simulink model "SF013A_PullCmpActv"  (R2013b)
settings: Solver=FixedStepDiscrete  SolverMode=SingleTasking  StartTime=0.0  StopTime=1  FixedStep=0.002  RelTol=1e-3
values from neighbouring files (symbols this model uses):
  ARCHGLBPRM_100MILLISEC_SEC_F32 = DataDict.Constant    [SF013A_PullCmpActv_DataDict.m]
  ARCHGLBPRM_2MILLISEC_SEC_F32 = DataDict.Constant    [SF013A_PullCmpActv_DataDict.m]
  ARCHGLBPRM_FLOATZEROTHD_ULS_F32 = DataDict.Constant    [SF013A_PullCmpActv_DataDict.m]
  INTGTRSCARSHOTERM_ULS_F32 = DataDict.Constant    [SF013A_PullCmpActv_DataDict.m]
  LONGTERMINTGTRSCAR_ULS_F32 = DataDict.Constant    [SF013A_PullCmpActv_DataDict.m]
  MICROSECTOSEC_ULS_F32 = DataDict.Constant    [SF013A_PullCmpActv_DataDict.m]
  MINSTOSEC_SECPERMINS_F32 = DataDict.Constant    [SF013A_PullCmpActv_DataDict.m]
  PullCmpActvCmpLrnTiDecShoTerm = DataDict.Calibration    [SF013A_PullCmpActv_DataDict.m]
  PullCmpActvCmpLrnTiIncShoTerm = DataDict.Calibration    [SF013A_PullCmpActv_DataDict.m]
  PullCmpActvCmpLrnTiLongTerm = DataDict.Calibration    [SF013A_PullCmpActv_DataDict.m]
  PullCmpActvCmpShoTermRstHwAgThd = DataDict.Calibration    [SF013A_PullCmpActv_DataDict.m]
  PullCmpActvCmpShoTermRstHwTqThd = DataDict.Calibration    [SF013A_PullCmpActv_DataDict.m]
  PullCmpActvCmpShoTermRstLatAThd = DataDict.Calibration    [SF013A_PullCmpActv_DataDict.m]
  PullCmpActvCmpShoTermRstYawRateThd = DataDict.Calibration    [SF013A_PullCmpActv_DataDict.m]
  PullCmpActvEna = DataDict.Calibration    [SF013A_PullCmpActv_DataDict.m]
  PullCmpActvLongTermLim = DataDict.Calibration    [SF013A_PullCmpActv_DataDict.m]
  PullCmpActvLrngEnaAgConfMinMgn = DataDict.Calibration    [SF013A_PullCmpActv_DataDict.m]
  PullCmpActvLrngEnaHwAgMaxMgn = DataDict.Calibration    [SF013A_PullCmpActv_DataDict.m]
  PullCmpActvLrngEnaHwTqMaxMgn = DataDict.Calibration    [SF013A_PullCmpActv_DataDict.m]
  PullCmpActvLrngEnaHwVelMaxMgn = DataDict.Calibration    [SF013A_PullCmpActv_DataDict.m]
  PullCmpActvLrngEnaLatAMaxMgn = DataDict.Calibration    [SF013A_PullCmpActv_DataDict.m]
  PullCmpActvLrngEnaTiThd = DataDict.Calibration    [SF013A_PullCmpActv_DataDict.m]
  PullCmpActvLrngEnaVehSpdMaxMgn = DataDict.Calibration    [SF013A_PullCmpActv_DataDict.m]
  PullCmpActvLrngEnaVehSpdMinMgn = DataDict.Calibration    [SF013A_PullCmpActv_DataDict.m]
  PullCmpActvLrngEnaVehSpdRateMaxMgn = DataDict.Calibration    [SF013A_PullCmpActv_DataDict.m]
  PullCmpActvLrngEnaYawRateMaxMgn = DataDict.Calibration    [SF013A_PullCmpActv_DataDict.m]
  PullCmpActvOpstSignTiShoTerm = DataDict.Calibration    [SF013A_PullCmpActv_DataDict.m]
  PullCmpActvOutpMaxRate = DataDict.Calibration    [SF013A_PullCmpActv_DataDict.m]
  PullCmpActvPullCmpShoTermLim = DataDict.Calibration    [SF013A_PullCmpActv_DataDict.m]
  PullCmpActvPullCmpTotLim = DataDict.Calibration    [SF013A_PullCmpActv_DataDict.m]
  PullCmpActvPullErrLimLongTerm = DataDict.Calibration    [SF013A_PullCmpActv_DataDict.m]
  PullCmpActvPullErrMgnThd = DataDict.Calibration    [SF013A_PullCmpActv_DataDict.m]
  PullCmpActvPullErrShoTermLim = DataDict.Calibration    [SF013A_PullCmpActv_DataDict.m]
  PullCmpActvShoTermRampTi = DataDict.Calibration    [SF013A_PullCmpActv_DataDict.m]
  SysGlbPrmSysTqRat = DataDict.ImprtdCal    [SF013A_PullCmpActv_DataDict.m]
libraries: NxtrAbslt x9, Fil x8, simulink x7, NxtrLim x6, FixdToFloat x3, NxtrSign x3, NxtrMin x3, NxtrNvM x2, NxtrMax x2, FloatToFixd x1, LnrIntrpn x1
(part 3 of 4)

== system SF013A_PullCmpActv/PullCmpActv/PullCmpActvPer1/PullCmpActvPer1/ActvCmpEna/ElapsedTime/If not true elapsed time = 0 ==
  Action Port : ActionPort  ActionType=then
  Constant : Constant  Value=0  OutDataTypeStr=single
  CopyRight2 : Subsystem  Description=|  mask(Copyright Information){none=on}
      | Copyright info block.                                               
      |                                                                     
      | Place copyright information at the top of every subsystem in design.
      mask prompts: none "No parameters"
      mask help: Place copyright information at the top of every subsystem in design.
      mask Display:
      | NxtrConf = 'Nexteer Confidential';
      | 
      | sys = bdroot; %handle for the current model ("system")
      | first = get_param(sys,'Created');
      | if(isempty(first))
      |     first = datestr(now,'yyyy');
      | else
      |     first = first(end-3:end);  %year is last four digits
      | end
      | 
      | last = get_param(sys,'LastModifiedDate');
      | if isempty(last)
      |     last = datestr(now,'yyyy');
      | else
      |     last = last(end-3:end);
      | end
      | 
      | if strcmp(first,last)
      |     fprintf('%s -- Copyright %s Nexteer',NxtrConf,first)
      | else
      |     fprintf('%s -- %s%s- %s Nexteer',NxtrConf,char(169),first,last)
      | end
  SpanTi : Outport
  wires:
  Constant/1 -> SpanTi/1

== system SF013A_PullCmpActv/PullCmpActv/PullCmpActvPer1/PullCmpActvPer1/ActvCmpEna/ElapsedTime/If true and last step is true calculate elapsed time  ==
  Action Port : ActionPort  ActionType=else
  Constant1 : Constant  Value=MICROSECTOSEC_ULS_F32
  CopyRight2 : Subsystem  Description=|  mask(Copyright Information){none=on}
      | Copyright info block.                                               
      |                                                                     
      | Place copyright information at the top of every subsystem in design.
      mask prompts: none "No parameters"
      mask help: Place copyright information at the top of every subsystem in design.
      mask Display:
      | NxtrConf = 'Nexteer Confidential';
      | 
      | sys = bdroot; %handle for the current model ("system")
      | first = get_param(sys,'Created');
      | if(isempty(first))
      |     first = datestr(now,'yyyy');
      | else
      |     first = first(end-3:end);  %year is last four digits
      | end
      | 
      | last = get_param(sys,'LastModifiedDate');
      | if isempty(last)
      |     last = datestr(now,'yyyy');
      | else
      |     last = last(end-3:end);
      | end
      | 
      | if strcmp(first,last)
      |     fprintf('%s -- Copyright %s Nexteer',NxtrConf,first)
      | else
      |     fprintf('%s -- %s%s- %s Nexteer',NxtrConf,char(169),first,last)
      | end
  Data Store Read : DataStoreRead  DataStoreName=RefTiEnaLrng
  Divide : Product  Inputs=**
  FixdToFloat_f32_u32 : FixdToFloat/FixdToFloat_f32_u32  Param1=0
  GetTiSpan100MicroSec32bit : Subsystem
  SpanTi : Outport
  wires:
  Constant1/1 -> Divide/2
  Divide/1 -> SpanTi/1
  GetTiSpan100MicroSec32bit/1(TiSpan) -> FixdToFloat_f32_u32/1
  Data Store Read/1 -> GetTiSpan100MicroSec32bit/1(RefTmr)
  FixdToFloat_f32_u32/1 -> Divide/1

== system SF013A_PullCmpActv/PullCmpActv/PullCmpActvPer1/PullCmpActvPer1/ActvCmpEna/ElapsedTime/If true and last step not true elapsed time = 0 get reference time  ==
  Action Port : ActionPort  ActionType=elseif
  Constant : Constant  Value=0  OutDataTypeStr=single
  CopyRight2 : Subsystem  Description=|  mask(Copyright Information){none=on}
      | Copyright info block.                                               
      |                                                                     
      | Place copyright information at the top of every subsystem in design.
      mask prompts: none "No parameters"
      mask help: Place copyright information at the top of every subsystem in design.
      mask Display:
      | NxtrConf = 'Nexteer Confidential';
      | 
      | sys = bdroot; %handle for the current model ("system")
      | first = get_param(sys,'Created');
      | if(isempty(first))
      |     first = datestr(now,'yyyy');
      | else
      |     first = first(end-3:end);  %year is last four digits
      | end
      | 
      | last = get_param(sys,'LastModifiedDate');
      | if isempty(last)
      |     last = datestr(now,'yyyy');
      | else
      |     last = last(end-3:end);
      | end
      | 
      | if strcmp(first,last)
      |     fprintf('%s -- Copyright %s Nexteer',NxtrConf,first)
      | else
      |     fprintf('%s -- %s%s- %s Nexteer',NxtrConf,char(169),first,last)
      | end
  Data Store Write : DataStoreWrite  DataStoreName=RefTiEnaLrng
  GetRefTmr100MicroSec32bit : Subsystem
  "SpanTi " : Outport
  wires:
  Constant/1 -> "SpanTi "/1
  GetRefTmr100MicroSec32bit/1(RefTmr) -> Data Store Write/1

== system SF013A_PullCmpActv/PullCmpActv/PullCmpActvPer1/PullCmpActvPer1/Calc_CmpTot/If Action Subsystem/CopyRight2 ==

== system SF013A_PullCmpActv/PullCmpActv/PullCmpActvPer1/PullCmpActvPer1/Calc_CmpTot/If Action Subsystem1/CopyRight2 ==

== system SF013A_PullCmpActv/PullCmpActv/PullCmpActvPer1/PullCmpActvPer1/ShoTermCmp/CalcIntgtrGain /CopyRight2 ==

== system SF013A_PullCmpActv/PullCmpActv/PullCmpActvPer1/PullCmpActvPer1/ShoTermCmp/CalcIntgtrGain /ElapsedTime ==
  note: If
  "OpstSign " : Inport
  CopyRight2 : Subsystem  Description=|  mask(Copyright Information){none=on}
      | Copyright info block.                                               
      |                                                                     
      | Place copyright information at the top of every subsystem in design.
      mask prompts: none "No parameters"
      mask help: Place copyright information at the top of every subsystem in design.
      mask Display:
      | NxtrConf = 'Nexteer Confidential';
      | 
      | sys = bdroot; %handle for the current model ("system")
      | first = get_param(sys,'Created');
      | if(isempty(first))
      |     first = datestr(now,'yyyy');
      | else
      |     first = first(end-3:end);  %year is last four digits
      | end
      | 
      | last = get_param(sys,'LastModifiedDate');
      | if isempty(last)
      |     last = datestr(now,'yyyy');
      | else
      |     last = last(end-3:end);
      | end
      | 
      | if strcmp(first,last)
      |     fprintf('%s -- Copyright %s Nexteer',NxtrConf,first)
      | else
      |     fprintf('%s -- %s%s- %s Nexteer',NxtrConf,char(169),first,last)
      | end
  Data Store Read : DataStoreRead  Priority=1  DataStoreName=OpstSignPrev
      settings: AttributesFormatString=priority: %<Priority>
  Data Store Write : DataStoreWrite  Priority=2  DataStoreName=OpstSignPrev
      settings: AttributesFormatString="priority:  %<Priority>"
  If : If  NumInputs=2  IfExpression=u1  ElseIfExpressions=u2
  If not true elapsed time = 0 : Subsystem  TreatAsAtomicUnit=on
  "If true and last step is true calculate elapsed time " : Subsystem  TreatAsAtomicUnit=on
  "If true and last step not true elapsed time = 0 get reference time " : Subsystem  TreatAsAtomicUnit=on
  Logical Operator : Logic  AllPortsSameDT=off  OutDataTypeStr=boolean
  Logical Operator1 : Logic  Operator=NOT  AllPortsSameDT=off  OutDataTypeStr=boolean
  Logical Operator2 : Logic  Operator=NOT  AllPortsSameDT=off  OutDataTypeStr=boolean
  Merge : Merge  Inputs=3
  ElapsedTime : Outport
  wires:
  If/1 -> If not true elapsed time = 0/Action
  If/2 -> "If true and last step not true elapsed time = 0 get reference time "/Action
  If/3 -> "If true and last step is true calculate elapsed time "/Action
  If not true elapsed time = 0/1(SpanTi) -> Merge/1
  "If true and last step not true elapsed time = 0 get reference time "/1("SpanTi ") -> Merge/2
  "If true and last step is true calculate elapsed time "/1(SpanTi) -> Merge/3
  Merge/1 -> ElapsedTime/1
  "OpstSign "/1 -> Logical Operator2/1, Logical Operator/1, Data Store Write/1
  Logical Operator1/1 -> Logical Operator/2
  Data Store Read/1 -> Logical Operator1/1
  Logical Operator/1 -> If/2
  Logical Operator2/1 -> If/1

== system SF013A_PullCmpActv/PullCmpActv/PullCmpActvPer1/PullCmpActvPer1/ShoTermCmp/CalcIntgtrGain /If Action Subsystem ==
  In1 : Inport
  Action Port : ActionPort  ActionType=then
  CopyRight2 : Subsystem  Description=|  mask(Copyright Information){none=on}
      | Copyright info block.                                               
      |                                                                     
      | Place copyright information at the top of every subsystem in design.
      mask prompts: none "No parameters"
      mask help: Place copyright information at the top of every subsystem in design.
      mask Display:
      | NxtrConf = 'Nexteer Confidential';
      | 
      | sys = bdroot; %handle for the current model ("system")
      | first = get_param(sys,'Created');
      | if(isempty(first))
      |     first = datestr(now,'yyyy');
      | else
      |     first = first(end-3:end);  %year is last four digits
      | end
      | 
      | last = get_param(sys,'LastModifiedDate');
      | if isempty(last)
      |     last = datestr(now,'yyyy');
      | else
      |     last = last(end-3:end);
      | end
      | 
      | if strcmp(first,last)
      |     fprintf('%s -- Copyright %s Nexteer',NxtrConf,first)
      | else
      |     fprintf('%s -- %s%s- %s Nexteer',NxtrConf,char(169),first,last)
      | end
  Out1 : Outport
  wires:
  In1/1 -> Out1/1

== system SF013A_PullCmpActv/PullCmpActv/PullCmpActvPer1/PullCmpActvPer1/ShoTermCmp/CalcIntgtrGain /If Action Subsystem1 ==
  In1 : Inport
  Action Port : ActionPort  ActionType=else
  CopyRight2 : Subsystem  Description=|  mask(Copyright Information){none=on}
      | Copyright info block.                                               
      |                                                                     
      | Place copyright information at the top of every subsystem in design.
      mask prompts: none "No parameters"
      mask help: Place copyright information at the top of every subsystem in design.
      mask Display:
      | NxtrConf = 'Nexteer Confidential';
      | 
      | sys = bdroot; %handle for the current model ("system")
      | first = get_param(sys,'Created');
      | if(isempty(first))
      |     first = datestr(now,'yyyy');
      | else
      |     first = first(end-3:end);  %year is last four digits
      | end
      | 
      | last = get_param(sys,'LastModifiedDate');
      | if isempty(last)
      |     last = datestr(now,'yyyy');
      | else
      |     last = last(end-3:end);
      | end
      | 
      | if strcmp(first,last)
      |     fprintf('%s -- Copyright %s Nexteer',NxtrConf,first)
      | else
      |     fprintf('%s -- %s%s- %s Nexteer',NxtrConf,char(169),first,last)
      | end
  Out1 : Outport
  wires:
  In1/1 -> Out1/1

== system SF013A_PullCmpActv/PullCmpActv/PullCmpActvPer1/PullCmpActvPer1/ShoTermCmp/CalcIntgtrGain /If Action Subsystem2 ==
  CmpLrnTi_Dec_ShoTerm : Inport
  Action Port : ActionPort  ActionType=then
  Constant3 : Constant  Value=INTGTRSCARSHOTERM_ULS_F32
  Constant4 : Constant  Value=ARCHGLBPRM_2MILLISEC_SEC_F32
  CopyRight2 : Subsystem  Description=|  mask(Copyright Information){none=on}
      | Copyright info block.                                               
      |                                                                     
      | Place copyright information at the top of every subsystem in design.
      mask prompts: none "No parameters"
      mask help: Place copyright information at the top of every subsystem in design.
      mask Display:
      | NxtrConf = 'Nexteer Confidential';
      | 
      | sys = bdroot; %handle for the current model ("system")
      | first = get_param(sys,'Created');
      | if(isempty(first))
      |     first = datestr(now,'yyyy');
      | else
      |     first = first(end-3:end);  %year is last four digits
      | end
      | 
      | last = get_param(sys,'LastModifiedDate');
      | if isempty(last)
      |     last = datestr(now,'yyyy');
      | else
      |     last = last(end-3:end);
      | end
      | 
      | if strcmp(first,last)
      |     fprintf('%s -- Copyright %s Nexteer',NxtrConf,first)
      | else
      |     fprintf('%s -- %s%s- %s Nexteer',NxtrConf,char(169),first,last)
      | end
  Data Store Write : DataStoreWrite  DataStoreName=IntgtrGainDecShoTerm
  Data Store Write1 : DataStoreWrite  DataStoreName=CmpLrnTiDecShoTerm
  Divide : Product  Inputs=*/
  Product : Product
  CmpIntglGain_Dec_ShoTerm : Outport
  wires:
  Constant3/1 -> Divide/1
  Product/1 -> CmpIntglGain_Dec_ShoTerm/1, Data Store Write/1
  Constant4/1 -> Product/1
  Divide/1 -> Product/2
  CmpLrnTi_Dec_ShoTerm/1 -> Data Store Write1/1, Divide/2

== system SF013A_PullCmpActv/PullCmpActv/PullCmpActvPer1/PullCmpActvPer1/ShoTermCmp/CalcIntgtrGain /If Action Subsystem3 ==
  In1 : Inport
  Action Port : ActionPort  ActionType=else
  CopyRight2 : Subsystem  Description=|  mask(Copyright Information){none=on}
      | Copyright info block.                                               
      |                                                                     
      | Place copyright information at the top of every subsystem in design.
      mask prompts: none "No parameters"
      mask help: Place copyright information at the top of every subsystem in design.
      mask Display:
      | NxtrConf = 'Nexteer Confidential';
      | 
      | sys = bdroot; %handle for the current model ("system")
      | first = get_param(sys,'Created');
      | if(isempty(first))
      |     first = datestr(now,'yyyy');
      | else
      |     first = first(end-3:end);  %year is last four digits
      | end
      | 
      | last = get_param(sys,'LastModifiedDate');
      | if isempty(last)
      |     last = datestr(now,'yyyy');
      | else
      |     last = last(end-3:end);
      | end
      | 
      | if strcmp(first,last)
      |     fprintf('%s -- Copyright %s Nexteer',NxtrConf,first)
      | else
      |     fprintf('%s -- %s%s- %s Nexteer',NxtrConf,char(169),first,last)
      | end
  Out1 : Outport
  wires:
  In1/1 -> Out1/1

== system SF013A_PullCmpActv/PullCmpActv/PullCmpActvPer1/PullCmpActvPer1/ShoTermCmp/CalcIntgtrGain /If Action Subsystem4 ==
  CmpLrnTi_Inc_ShoTerm : Inport
  Action Port : ActionPort  ActionType=then
  Constant3 : Constant  Value=INTGTRSCARSHOTERM_ULS_F32
  Constant4 : Constant  Value=ARCHGLBPRM_2MILLISEC_SEC_F32
  CopyRight2 : Subsystem  Description=|  mask(Copyright Information){none=on}
      | Copyright info block.                                               
      |                                                                     
      | Place copyright information at the top of every subsystem in design.
      mask prompts: none "No parameters"
      mask help: Place copyright information at the top of every subsystem in design.
      mask Display:
      | NxtrConf = 'Nexteer Confidential';
      | 
      | sys = bdroot; %handle for the current model ("system")
      | first = get_param(sys,'Created');
      | if(isempty(first))
      |     first = datestr(now,'yyyy');
      | else
      |     first = first(end-3:end);  %year is last four digits
      | end
      | 
      | last = get_param(sys,'LastModifiedDate');
      | if isempty(last)
      |     last = datestr(now,'yyyy');
      | else
      |     last = last(end-3:end);
      | end
      | 
      | if strcmp(first,last)
      |     fprintf('%s -- Copyright %s Nexteer',NxtrConf,first)
      | else
      |     fprintf('%s -- %s%s- %s Nexteer',NxtrConf,char(169),first,last)
      | end
  Data Store Write : DataStoreWrite  DataStoreName=CmpLrnTiIncShoTerm
  Data Store Write1 : DataStoreWrite  DataStoreName=IntgtrGainIncShoTerm
  Divide : Product  Inputs=*/
  Product : Product
  CmpIntglGain_Inc_ShoTerm : Outport
  wires:
  CmpLrnTi_Inc_ShoTerm/1 -> Data Store Write/1, Divide/2
  Divide/1 -> Product/2
  Constant4/1 -> Product/1
  Constant3/1 -> Divide/1
  Product/1 -> CmpIntglGain_Inc_ShoTerm/1, Data Store Write1/1

== system SF013A_PullCmpActv/PullCmpActv/PullCmpActvPer1/PullCmpActvPer1/ShoTermCmp/CalcIntgtrGain /If Action Subsystem5 ==
  In1 : Inport
  Action Port : ActionPort  ActionType=else
  CopyRight2 : Subsystem  Description=|  mask(Copyright Information){none=on}
      | Copyright info block.                                               
      |                                                                     
      | Place copyright information at the top of every subsystem in design.
      mask prompts: none "No parameters"
      mask help: Place copyright information at the top of every subsystem in design.
      mask Display:
      | NxtrConf = 'Nexteer Confidential';
      | 
      | sys = bdroot; %handle for the current model ("system")
      | first = get_param(sys,'Created');
      | if(isempty(first))
      |     first = datestr(now,'yyyy');
      | else
      |     first = first(end-3:end);  %year is last four digits
      | end
      | 
      | last = get_param(sys,'LastModifiedDate');
      | if isempty(last)
      |     last = datestr(now,'yyyy');
      | else
      |     last = last(end-3:end);
      | end
      | 
      | if strcmp(first,last)
      |     fprintf('%s -- Copyright %s Nexteer',NxtrConf,first)
      | else
      |     fprintf('%s -- %s%s- %s Nexteer',NxtrConf,char(169),first,last)
      | end
  Out1 : Outport
  wires:
  In1/1 -> Out1/1

== system SF013A_PullCmpActv/PullCmpActv/PullCmpActvPer1/PullCmpActvPer1/ShoTermCmp/ErrIntgtr & ActvLim /CopyRight2 ==

== system SF013A_PullCmpActv/PullCmpActv/PullCmpActvPer1/PullCmpActvPer1/ShoTermCmp/ErrIntgtr & ActvLim /If Action Subsystem2 ==
  In1 : Inport
  Action Port : ActionPort  ActionType=then
  CopyRight2 : Subsystem  Description=|  mask(Copyright Information){none=on}
      | Copyright info block.                                               
      |                                                                     
      | Place copyright information at the top of every subsystem in design.
      mask prompts: none "No parameters"
      mask help: Place copyright information at the top of every subsystem in design.
      mask Display:
      | NxtrConf = 'Nexteer Confidential';
      | 
      | sys = bdroot; %handle for the current model ("system")
      | first = get_param(sys,'Created');
      | if(isempty(first))
      |     first = datestr(now,'yyyy');
      | else
      |     first = first(end-3:end);  %year is last four digits
      | end
      | 
      | last = get_param(sys,'LastModifiedDate');
      | if isempty(last)
      |     last = datestr(now,'yyyy');
      | else
      |     last = last(end-3:end);
      | end
      | 
      | if strcmp(first,last)
      |     fprintf('%s -- Copyright %s Nexteer',NxtrConf,first)
      | else
      |     fprintf('%s -- %s%s- %s Nexteer',NxtrConf,char(169),first,last)
      | end
  Out1 : Outport
  wires:
  In1/1 -> Out1/1

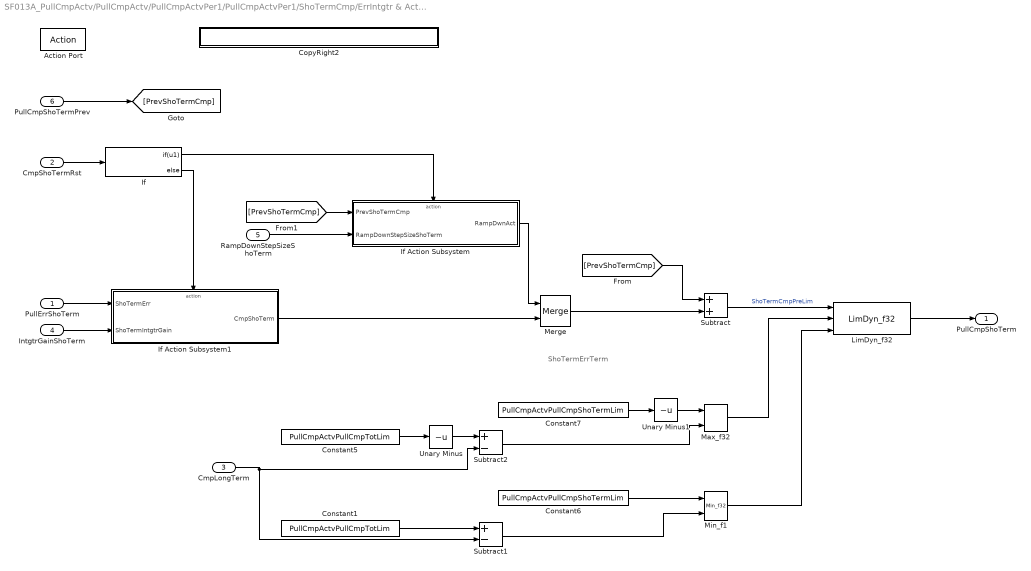
== system SF013A_PullCmpActv/PullCmpActv/PullCmpActvPer1/PullCmpActvPer1/ShoTermCmp/ErrIntgtr & ActvLim /If Action Subsystem3 ==
  note: ShoTermErrTerm
  PullErrShoTerm : Inport
  "CmpShoTermRst " : Inport  Port=2
  CmpLongTerm : Inport  Port=3
  IntgtrGainShoTerm : Inport  Port=4
  RampDownStepSizeShoTerm : Inport  Port=5
  PullCmpShoTermPrev : Inport  Port=6
  Action Port : ActionPort  ActionType=else
  Constant1 : Constant  Value=PullCmpActvPullCmpTotLim
  Constant5 : Constant  Value=PullCmpActvPullCmpTotLim
  Constant6 : Constant  Value=PullCmpActvPullCmpShoTermLim
  Constant7 : Constant  Value=PullCmpActvPullCmpShoTermLim
  CopyRight2 : Subsystem  Description=|  mask(Copyright Information){none=on}
      | Copyright info block.                                               
      |                                                                     
      | Place copyright information at the top of every subsystem in design.
      mask prompts: none "No parameters"
      mask help: Place copyright information at the top of every subsystem in design.
      mask Display:
      | NxtrConf = 'Nexteer Confidential';
      | 
      | sys = bdroot; %handle for the current model ("system")
      | first = get_param(sys,'Created');
      | if(isempty(first))
      |     first = datestr(now,'yyyy');
      | else
      |     first = first(end-3:end);  %year is last four digits
      | end
      | 
      | last = get_param(sys,'LastModifiedDate');
      | if isempty(last)
      |     last = datestr(now,'yyyy');
      | else
      |     last = last(end-3:end);
      | end
      | 
      | if strcmp(first,last)
      |     fprintf('%s -- Copyright %s Nexteer',NxtrConf,first)
      | else
      |     fprintf('%s -- %s%s- %s Nexteer',NxtrConf,char(169),first,last)
      | end
  If : If  IfExpression=u1
  If Action Subsystem : Subsystem  TreatAsAtomicUnit=on
  If Action Subsystem1 : Subsystem  TreatAsAtomicUnit=on
  LimDyn_f32 : NxtrLim/LimDyn_f32
  Max_f32 : NxtrMax/Max_f32  SFunctionSpec=single y1 = Max_f32(single u1, single u2)
      settings: AttributesFormatString=%<Name>
  Merge : Merge
  Min_f1 : NxtrMin/Min_f32  SFunctionSpec=single y1 = Min_f32(single u1, single u2)
      settings: AttributesFormatString=%<Name>
  Subtract : Sum
  Subtract1 : Sum  Inputs=+-
  Subtract2 : Sum  Inputs=+-
  Unary Minus : UnaryMinus
  Unary Minus1 : UnaryMinus
  PullCmpShoTerm : Outport
  wires:
  "CmpShoTermRst "/1 -> If/1
  Merge/1 -> Subtract/2
  Subtract/1 -> LimDyn_f32/1  "ShoTermCmpPreLim"
  Constant1/1 -> Subtract1/1
  CmpLongTerm/1 -> Subtract1/2, Subtract2/2
  Constant5/1 -> Unary Minus/1
  Unary Minus/1 -> Subtract2/1
  Constant6/1 -> Min_f1/1
  Subtract1/1 -> Min_f1/2
  Constant7/1 -> Unary Minus1/1
  Unary Minus1/1 -> Max_f32/1
  Subtract2/1 -> Max_f32/2
  Max_f32/1 -> LimDyn_f32/2
  Min_f1/1 -> LimDyn_f32/3
  If/1 -> If Action Subsystem/Action
  [PrevShoTermCmp] -> If Action Subsystem/1(PrevShoTermCmp)
  RampDownStepSizeShoTerm/1 -> If Action Subsystem/2(RampDownStepSizeShoTerm)
  If/2 -> If Action Subsystem1/Action
  PullErrShoTerm/1 -> If Action Subsystem1/1(ShoTermErr)
  IntgtrGainShoTerm/1 -> If Action Subsystem1/2(ShoTermIntgtrGain)
  If Action Subsystem/1(RampDwnAct) -> Merge/1
  If Action Subsystem1/1(CmpShoTerm) -> Merge/2
  [PrevShoTermCmp] -> Subtract/1
  LimDyn_f32/1 -> PullCmpShoTerm/1
  PullCmpShoTermPrev/1 -> [PrevShoTermCmp]

== system SF013A_PullCmpActv/PullCmpActv/PullCmpActvPer1/PullCmpActvPer1/ShoTermCmp/ShoTermCmpFil/CopyRight2 ==

== system SF013A_PullCmpActv/PullCmpActv/PullCmpActvPer1/PullCmpActvPer1/ShoTermCmp/ShoTermCmpFil/If Action Subsystem ==
  In1 : Inport
  Action Port : ActionPort  ActionType=then
  CopyRight2 : Subsystem  Description=|  mask(Copyright Information){none=on}
      | Copyright info block.                                               
      |                                                                     
      | Place copyright information at the top of every subsystem in design.
      mask prompts: none "No parameters"
      mask help: Place copyright information at the top of every subsystem in design.
      mask Display:
      | NxtrConf = 'Nexteer Confidential';
      | 
      | sys = bdroot; %handle for the current model ("system")
      | first = get_param(sys,'Created');
      | if(isempty(first))
      |     first = datestr(now,'yyyy');
      | else
      |     first = first(end-3:end);  %year is last four digits
      | end
      | 
      | last = get_param(sys,'LastModifiedDate');
      | if isempty(last)
      |     last = datestr(now,'yyyy');
      | else
      |     last = last(end-3:end);
      | end
      | 
      | if strcmp(first,last)
      |     fprintf('%s -- Copyright %s Nexteer',NxtrConf,first)
      | else
      |     fprintf('%s -- %s%s- %s Nexteer',NxtrConf,char(169),first,last)
      | end
  Out1 : Outport
  wires:
  In1/1 -> Out1/1

== system SF013A_PullCmpActv/PullCmpActv/PullCmpActvPer1/PullCmpActvPer1/ShoTermCmp/ShoTermCmpFil/If Action Subsystem1 ==
  In1 : Inport
  Action Port : ActionPort  ActionType=else
  CopyRight2 : Subsystem  Description=|  mask(Copyright Information){none=on}
      | Copyright info block.                                               
      |                                                                     
      | Place copyright information at the top of every subsystem in design.
      mask prompts: none "No parameters"
      mask help: Place copyright information at the top of every subsystem in design.
      mask Display:
      | NxtrConf = 'Nexteer Confidential';
      | 
      | sys = bdroot; %handle for the current model ("system")
      | first = get_param(sys,'Created');
      | if(isempty(first))
      |     first = datestr(now,'yyyy');
      | else
      |     first = first(end-3:end);  %year is last four digits
      | end
      | 
      | last = get_param(sys,'LastModifiedDate');
      | if isempty(last)
      |     last = datestr(now,'yyyy');
      | else
      |     last = last(end-3:end);
      | end
      | 
      | if strcmp(first,last)
      |     fprintf('%s -- Copyright %s Nexteer',NxtrConf,first)
      | else
      |     fprintf('%s -- %s%s- %s Nexteer',NxtrConf,char(169),first,last)
      | end
  Out1 : Outport
  wires:
  In1/1 -> Out1/1

== system SF013A_PullCmpActv/PullCmpActv/PullCmpActvPer2/PullCmpActvPer2/LongTermCmpFil/If Action Subsystem/CopyRight2 ==

== system SF013A_PullCmpActv/PullCmpActv/PullCmpActvPer2/PullCmpActvPer2/LongTermCmpFil/If Action Subsystem1/CopyRight2 ==

== system SF013A_PullCmpActv/PullCmpActv/PullCmpActvPer2/PullCmpActvPer2/LongTermErrIntgtr /If Action Subsystem/CopyRight2 ==

== system SF013A_PullCmpActv/PullCmpActv/PullCmpActvPer2/PullCmpActvPer2/LongTermErrIntgtr /If Action Subsystem1/CopyRight2 ==

== system SF013A_PullCmpActv/PullCmpActv/PullCmpActvPer2/PullCmpActvPer2/LongTermErrIntgtr /If Action Subsystem1/If Action Subsystem ==
  In2 : Inport
  Action Port : ActionPort  ActionType=then
  Constant1 : Constant  Value=MINSTOSEC_SECPERMINS_F32
  Constant3 : Constant  Value=LONGTERMINTGTRSCAR_ULS_F32
  Constant4 : Constant  Value=ARCHGLBPRM_100MILLISEC_SEC_F32
  CopyRight2 : Subsystem  Description=|  mask(Copyright Information){none=on}
      | Copyright info block.                                               
      |                                                                     
      | Place copyright information at the top of every subsystem in design.
      mask prompts: none "No parameters"
      mask help: Place copyright information at the top of every subsystem in design.
      mask Display:
      | NxtrConf = 'Nexteer Confidential';
      | 
      | sys = bdroot; %handle for the current model ("system")
      | first = get_param(sys,'Created');
      | if(isempty(first))
      |     first = datestr(now,'yyyy');
      | else
      |     first = first(end-3:end);  %year is last four digits
      | end
      | 
      | last = get_param(sys,'LastModifiedDate');
      | if isempty(last)
      |     last = datestr(now,'yyyy');
      | else
      |     last = last(end-3:end);
      | end
      | 
      | if strcmp(first,last)
      |     fprintf('%s -- Copyright %s Nexteer',NxtrConf,first)
      | else
      |     fprintf('%s -- %s%s- %s Nexteer',NxtrConf,char(169),first,last)
      | end
  Data Store Write : DataStoreWrite  DataStoreName=CmpLrnTiLongTerm
  Divide : Product  Inputs=**//
  LrnTiLongTerm : Outport
  wires:
  Constant4/1 -> Divide/1
  Divide/1 -> Data Store Write/1, LrnTiLongTerm/1
  Constant1/1 -> Divide/4
  Constant3/1 -> Divide/2
  In2/1 -> Divide/3

== system SF013A_PullCmpActv/PullCmpActv/PullCmpActvPer2/PullCmpActvPer2/LongTermErrIntgtr /If Action Subsystem1/If Action Subsystem1 ==
  In1 : Inport
  Action Port : ActionPort  ActionType=else
  CopyRight2 : Subsystem  Description=|  mask(Copyright Information){none=on}
      | Copyright info block.                                               
      |                                                                     
      | Place copyright information at the top of every subsystem in design.
      mask prompts: none "No parameters"
      mask help: Place copyright information at the top of every subsystem in design.
      mask Display:
      | NxtrConf = 'Nexteer Confidential';
      | 
      | sys = bdroot; %handle for the current model ("system")
      | first = get_param(sys,'Created');
      | if(isempty(first))
      |     first = datestr(now,'yyyy');
      | else
      |     first = first(end-3:end);  %year is last four digits
      | end
      | 
      | last = get_param(sys,'LastModifiedDate');
      | if isempty(last)
      |     last = datestr(now,'yyyy');
      | else
      |     last = last(end-3:end);
      | end
      | 
      | if strcmp(first,last)
      |     fprintf('%s -- Copyright %s Nexteer',NxtrConf,first)
      | else
      |     fprintf('%s -- %s%s- %s Nexteer',NxtrConf,char(169),first,last)
      | end
  LrnTiLongTerm : Outport
  wires:
  In1/1 -> LrnTiLongTerm/1

== system SF013A_PullCmpActv/PullCmpActv/PullCmpActvPer1/PullCmpActvPer1/ActvCmpEna/ElapsedTime/If not true elapsed time = 0/CopyRight2 ==

== system SF013A_PullCmpActv/PullCmpActv/PullCmpActvPer1/PullCmpActvPer1/ActvCmpEna/ElapsedTime/If true and last step is true calculate elapsed time /CopyRight2 ==

== system SF013A_PullCmpActv/PullCmpActv/PullCmpActvPer1/PullCmpActvPer1/ActvCmpEna/ElapsedTime/If true and last step is true calculate elapsed time /GetTiSpan100MicroSec32bit ==
  note: Subtract original reference time
  note: seconds
  note: microseconds
  note: counts
  note: Wrap-to-zero
  note: 1 count = 100 uSec
  note: Get current system time
  note: GetTiSpan100MicroSec32bit
  RefTmr : Inport
  CopyRight2 : Subsystem  Description=|  mask(Copyright Information){none=on}
      | Copyright info block.                                               
      |                                                                     
      | Place copyright information at the top of every subsystem in design.
      mask prompts: none "No parameters"
      mask help: Place copyright information at the top of every subsystem in design.
      mask Display:
      | NxtrConf = 'Nexteer Confidential';
      | 
      | sys = bdroot; %handle for the current model ("system")
      | first = get_param(sys,'Created');
      | if(isempty(first))
      |     first = datestr(now,'yyyy');
      | else
      |     first = first(end-3:end);  %year is last four digits
      | end
      | 
      | last = get_param(sys,'LastModifiedDate');
      | if isempty(last)
      |     last = datestr(now,'yyyy');
      | else
      |     last = last(end-3:end);
      | end
      | 
      | if strcmp(first,last)
      |     fprintf('%s -- Copyright %s Nexteer',NxtrConf,first)
      | else
      |     fprintf('%s -- %s%s- %s Nexteer',NxtrConf,char(169),first,last)
      | end
  Count per uSec : Constant  Value=0.01
  Data Store Read1 : DataStoreRead  DataStoreName=SimnTi
  Data Type Conversion2 : DataTypeConversion  OutDataTypeStr=uint32
  Divide1 : Product  Inputs=**
  Divide2 : Product  Inputs=*/
  If : If  NumInputs=2  IfExpression=u1 >= u2
  Max Counts : Constant  Value=2^32-1
  Merge : Merge
  No wrapping : Subsystem  TreatAsAtomicUnit=on
  Product2 : Product
  Product3 : Product
  Rounding : Rounding
  Subtract3 : Sum  Inputs=+-
  Wrapping : Subsystem  TreatAsAtomicUnit=on
  uSec per Sec : Constant  Value=1000000
  TiSpan : Outport
  wires:
  Wrapping/1(Out1) -> Merge/2
  No wrapping/1(Out1) -> Merge/1
  If/2 -> Wrapping/Action
  If/1 -> No wrapping/Action
  Product3/1 -> Subtract3/2
  Subtract3/1 -> Data Type Conversion2/1
  Rounding/1 -> Product3/1
  Divide2/1 -> Rounding/1
  Max Counts/1 -> Divide2/2, Product3/2
  Divide1/1 -> Divide2/1, Subtract3/1
  Product2/1 -> Divide1/1
  Data Store Read1/1 -> Product2/1
  Count per uSec/1 -> Divide1/2
  uSec per Sec/1 -> Product2/2
  Merge/1 -> TiSpan/1
  RefTmr/1 -> If/2, No wrapping/2(ref), Wrapping/2(ref)
  Data Type Conversion2/1 -> If/1, No wrapping/1(new), Wrapping/1(new)

== system SF013A_PullCmpActv/PullCmpActv/PullCmpActvPer1/PullCmpActvPer1/ActvCmpEna/ElapsedTime/If true and last step not true elapsed time = 0 get reference time /CopyRight2 ==

== system SF013A_PullCmpActv/PullCmpActv/PullCmpActvPer1/PullCmpActvPer1/ActvCmpEna/ElapsedTime/If true and last step not true elapsed time = 0 get reference time /GetRefTmr100MicroSec32bit ==
  note: 1 count = 100 uSec
  note: seconds
  note: microseconds
  note: counts
  note: Wrap-to-zero
  note: GetRefTmr100MicroSec32bit
  CopyRight2 : Subsystem  Description=|  mask(Copyright Information){none=on}
      | Copyright info block.                                               
      |                                                                     
      | Place copyright information at the top of every subsystem in design.
      mask prompts: none "No parameters"
      mask help: Place copyright information at the top of every subsystem in design.
      mask Display:
      | NxtrConf = 'Nexteer Confidential';
      | 
      | sys = bdroot; %handle for the current model ("system")
      | first = get_param(sys,'Created');
      | if(isempty(first))
      |     first = datestr(now,'yyyy');
      | else
      |     first = first(end-3:end);  %year is last four digits
      | end
      | 
      | last = get_param(sys,'LastModifiedDate');
      | if isempty(last)
      |     last = datestr(now,'yyyy');
      | else
      |     last = last(end-3:end);
      | end
      | 
      | if strcmp(first,last)
      |     fprintf('%s -- Copyright %s Nexteer',NxtrConf,first)
      | else
      |     fprintf('%s -- %s%s- %s Nexteer',NxtrConf,char(169),first,last)
      | end
  Count per uSec : Constant  Value=0.01
  Data Store Read1 : DataStoreRead  DataStoreName=SimnTi
  Data Type Conversion1 : DataTypeConversion  OutDataTypeStr=uint32
  Divide1 : Product  Inputs=**
  Divide2 : Product  Inputs=*/
  Max Counts : Constant  Value=2^32-1
  Product1 : Product
  Product2 : Product
  Rounding : Rounding
  Subtract1 : Sum  Inputs=+-
  uSec per Sec : Constant  Value=1000000
  RefTmr : Outport
  wires:
  Product2/1 -> Subtract1/2
  Subtract1/1 -> Data Type Conversion1/1
  Rounding/1 -> Product2/1
  Divide2/1 -> Rounding/1
  Max Counts/1 -> Divide2/2, Product2/2
  Divide1/1 -> Divide2/1, Subtract1/1
  Product1/1 -> Divide1/1
  Data Store Read1/1 -> Product1/1
  Count per uSec/1 -> Divide1/2
  uSec per Sec/1 -> Product1/2
  Data Type Conversion1/1 -> RefTmr/1

== system SF013A_PullCmpActv/PullCmpActv/PullCmpActvPer1/PullCmpActvPer1/ShoTermCmp/CalcIntgtrGain /ElapsedTime/CopyRight2 ==

== system SF013A_PullCmpActv/PullCmpActv/PullCmpActvPer1/PullCmpActvPer1/ShoTermCmp/CalcIntgtrGain /ElapsedTime/If not true elapsed time = 0 ==
  Action Port : ActionPort  ActionType=then
  Constant : Constant  Value=0  OutDataTypeStr=single
  CopyRight2 : Subsystem  Description=|  mask(Copyright Information){none=on}
      | Copyright info block.                                               
      |                                                                     
      | Place copyright information at the top of every subsystem in design.
      mask prompts: none "No parameters"
      mask help: Place copyright information at the top of every subsystem in design.
      mask Display:
      | NxtrConf = 'Nexteer Confidential';
      | 
      | sys = bdroot; %handle for the current model ("system")
      | first = get_param(sys,'Created');
      | if(isempty(first))
      |     first = datestr(now,'yyyy');
      | else
      |     first = first(end-3:end);  %year is last four digits
      | end
      | 
      | last = get_param(sys,'LastModifiedDate');
      | if isempty(last)
      |     last = datestr(now,'yyyy');
      | else
      |     last = last(end-3:end);
      | end
      | 
      | if strcmp(first,last)
      |     fprintf('%s -- Copyright %s Nexteer',NxtrConf,first)
      | else
      |     fprintf('%s -- %s%s- %s Nexteer',NxtrConf,char(169),first,last)
      | end
  SpanTi : Outport
  wires:
  Constant/1 -> SpanTi/1

== system SF013A_PullCmpActv/PullCmpActv/PullCmpActvPer1/PullCmpActvPer1/ShoTermCmp/CalcIntgtrGain /ElapsedTime/If true and last step is true calculate elapsed time  ==
  Action Port : ActionPort  ActionType=else
  Constant1 : Constant  Value=MICROSECTOSEC_ULS_F32
  CopyRight2 : Subsystem  Description=|  mask(Copyright Information){none=on}
      | Copyright info block.                                               
      |                                                                     
      | Place copyright information at the top of every subsystem in design.
      mask prompts: none "No parameters"
      mask help: Place copyright information at the top of every subsystem in design.
      mask Display:
      | NxtrConf = 'Nexteer Confidential';
      | 
      | sys = bdroot; %handle for the current model ("system")
      | first = get_param(sys,'Created');
      | if(isempty(first))
      |     first = datestr(now,'yyyy');
      | else
      |     first = first(end-3:end);  %year is last four digits
      | end
      | 
      | last = get_param(sys,'LastModifiedDate');
      | if isempty(last)
      |     last = datestr(now,'yyyy');
      | else
      |     last = last(end-3:end);
      | end
      | 
      | if strcmp(first,last)
      |     fprintf('%s -- Copyright %s Nexteer',NxtrConf,first)
      | else
      |     fprintf('%s -- %s%s- %s Nexteer',NxtrConf,char(169),first,last)
      | end
  Data Store Read : DataStoreRead  DataStoreName=RefTiOpstSign
  Divide : Product  Inputs=**
  FixdToFloat_f32_u32 : FixdToFloat/FixdToFloat_f32_u32  Param1=0
  GetTiSpan100MicroSec32bit : Subsystem
  SpanTi : Outport
  wires:
  Constant1/1 -> Divide/2
  Divide/1 -> SpanTi/1
  GetTiSpan100MicroSec32bit/1(TiSpan) -> FixdToFloat_f32_u32/1
  Data Store Read/1 -> GetTiSpan100MicroSec32bit/1(RefTmr)
  FixdToFloat_f32_u32/1 -> Divide/1

== system SF013A_PullCmpActv/PullCmpActv/PullCmpActvPer1/PullCmpActvPer1/ShoTermCmp/CalcIntgtrGain /ElapsedTime/If true and last step not true elapsed time = 0 get reference time  ==
  Action Port : ActionPort  ActionType=elseif
  Constant : Constant  Value=0  OutDataTypeStr=single
  CopyRight2 : Subsystem  Description=|  mask(Copyright Information){none=on}
      | Copyright info block.                                               
      |                                                                     
      | Place copyright information at the top of every subsystem in design.
      mask prompts: none "No parameters"
      mask help: Place copyright information at the top of every subsystem in design.
      mask Display:
      | NxtrConf = 'Nexteer Confidential';
      | 
      | sys = bdroot; %handle for the current model ("system")
      | first = get_param(sys,'Created');
      | if(isempty(first))
      |     first = datestr(now,'yyyy');
      | else
      |     first = first(end-3:end);  %year is last four digits
      | end
      | 
      | last = get_param(sys,'LastModifiedDate');
      | if isempty(last)
      |     last = datestr(now,'yyyy');
      | else
      |     last = last(end-3:end);
      | end
      | 
      | if strcmp(first,last)
      |     fprintf('%s -- Copyright %s Nexteer',NxtrConf,first)
      | else
      |     fprintf('%s -- %s%s- %s Nexteer',NxtrConf,char(169),first,last)
      | end
  Data Store Write : DataStoreWrite  DataStoreName=RefTiOpstSign
  GetRefTmr100MicroSec32bit : Subsystem
  "SpanTi " : Outport
  wires:
  Constant/1 -> "SpanTi "/1
  GetRefTmr100MicroSec32bit/1(RefTmr) -> Data Store Write/1

== system SF013A_PullCmpActv/PullCmpActv/PullCmpActvPer1/PullCmpActvPer1/ShoTermCmp/CalcIntgtrGain /If Action Subsystem/CopyRight2 ==

== system SF013A_PullCmpActv/PullCmpActv/PullCmpActvPer1/PullCmpActvPer1/ShoTermCmp/CalcIntgtrGain /If Action Subsystem1/CopyRight2 ==

== system SF013A_PullCmpActv/PullCmpActv/PullCmpActvPer1/PullCmpActvPer1/ShoTermCmp/CalcIntgtrGain /If Action Subsystem2/CopyRight2 ==

== system SF013A_PullCmpActv/PullCmpActv/PullCmpActvPer1/PullCmpActvPer1/ShoTermCmp/CalcIntgtrGain /If Action Subsystem3/CopyRight2 ==

== system SF013A_PullCmpActv/PullCmpActv/PullCmpActvPer1/PullCmpActvPer1/ShoTermCmp/CalcIntgtrGain /If Action Subsystem4/CopyRight2 ==

== system SF013A_PullCmpActv/PullCmpActv/PullCmpActvPer1/PullCmpActvPer1/ShoTermCmp/CalcIntgtrGain /If Action Subsystem5/CopyRight2 ==

== system SF013A_PullCmpActv/PullCmpActv/PullCmpActvPer1/PullCmpActvPer1/ShoTermCmp/ErrIntgtr & ActvLim /If Action Subsystem2/CopyRight2 ==

== system SF013A_PullCmpActv/PullCmpActv/PullCmpActvPer1/PullCmpActvPer1/ShoTermCmp/ErrIntgtr & ActvLim /If Action Subsystem3/CopyRight2 ==

== system SF013A_PullCmpActv/PullCmpActv/PullCmpActvPer1/PullCmpActvPer1/ShoTermCmp/ErrIntgtr & ActvLim /If Action Subsystem3/If Action Subsystem ==
  PrevShoTermCmp : Inport
  RampDownStepSizeShoTerm : Inport  Port=2
  Action Port : ActionPort  ActionType=then
  Abslt_f32_f32 : NxtrAbslt/Abslt_f32_f32  SFunctionSpec=single y1 = Abslt_f32_f32(single u1)
      settings: AttributesFormatString=%<Name>
  CopyRight2 : Subsystem  Description=|  mask(Copyright Information){none=on}
      | Copyright info block.                                               
      |                                                                     
      | Place copyright information at the top of every subsystem in design.
      mask prompts: none "No parameters"
      mask help: Place copyright information at the top of every subsystem in design.
      mask Display:
      | NxtrConf = 'Nexteer Confidential';
      | 
      | sys = bdroot; %handle for the current model ("system")
      | first = get_param(sys,'Created');
      | if(isempty(first))
      |     first = datestr(now,'yyyy');
      | else
      |     first = first(end-3:end);  %year is last four digits
      | end
      | 
      | last = get_param(sys,'LastModifiedDate');
      | if isempty(last)
      |     last = datestr(now,'yyyy');
      | else
      |     last = last(end-3:end);
      | end
      | 
      | if strcmp(first,last)
      |     fprintf('%s -- Copyright %s Nexteer',NxtrConf,first)
      | else
      |     fprintf('%s -- %s%s- %s Nexteer',NxtrConf,char(169),first,last)
      | end
  Min_f32 : NxtrMin/Min_f32  SFunctionSpec=single y1 = Min_f32(single u1, single u2)
      settings: AttributesFormatString=%<Name>
  Product1 : Product
  Sign_s08_f32 : NxtrSign/Sign_s08_f32  SFunctionSpec=int8 y1 = Sign_s08_f32(single u1)
  Unary Minus2 : UnaryMinus
  RampDwnAct : Outport
  wires:
  PrevShoTermCmp/1 -> Sign_s08_f32/1, Abslt_f32_f32/1
  Abslt_f32_f32/1 -> Min_f32/1
  RampDownStepSizeShoTerm/1 -> Min_f32/2
  Sign_s08_f32/1 -> Unary Minus2/1
  Unary Minus2/1 -> Product1/1
  Min_f32/1 -> Product1/2
  Product1/1 -> RampDwnAct/1

== system SF013A_PullCmpActv/PullCmpActv/PullCmpActvPer1/PullCmpActvPer1/ShoTermCmp/ErrIntgtr & ActvLim /If Action Subsystem3/If Action Subsystem1 ==
  ShoTermErr : Inport
  ShoTermIntgtrGain : Inport  Port=2
  Action Port : ActionPort  ActionType=else
  Constant : Constant  Value=PullCmpActvPullErrShoTermLim
  CopyRight2 : Subsystem  Description=|  mask(Copyright Information){none=on}
      | Copyright info block.                                               
      |                                                                     
      | Place copyright information at the top of every subsystem in design.
      mask prompts: none "No parameters"
      mask help: Place copyright information at the top of every subsystem in design.
      mask Display:
      | NxtrConf = 'Nexteer Confidential';
      | 
      | sys = bdroot; %handle for the current model ("system")
      | first = get_param(sys,'Created');
      | if(isempty(first))
      |     first = datestr(now,'yyyy');
      | else
      |     first = first(end-3:end);  %year is last four digits
      | end
      | 
      | last = get_param(sys,'LastModifiedDate');
      | if isempty(last)
      |     last = datestr(now,'yyyy');
      | else
      |     last = last(end-3:end);
      | end
      | 
      | if strcmp(first,last)
      |     fprintf('%s -- Copyright %s Nexteer',NxtrConf,first)
      | else
      |     fprintf('%s -- %s%s- %s Nexteer',NxtrConf,char(169),first,last)
      | end
  LimDyn_f32 : NxtrLim/LimDyn_f32
  Product : Product
  Unary Minus : UnaryMinus
  CmpShoTerm : Outport
  wires:
  ShoTermErr/1 -> LimDyn_f32/1
  LimDyn_f32/1 -> Product/2
  ShoTermIntgtrGain/1 -> Product/1
  Product/1 -> CmpShoTerm/1
  Constant/1 -> Unary Minus/1, LimDyn_f32/3
  Unary Minus/1 -> LimDyn_f32/2

== system SF013A_PullCmpActv/PullCmpActv/PullCmpActvPer1/PullCmpActvPer1/ShoTermCmp/ShoTermCmpFil/If Action Subsystem/CopyRight2 ==

== system SF013A_PullCmpActv/PullCmpActv/PullCmpActvPer1/PullCmpActvPer1/ShoTermCmp/ShoTermCmpFil/If Action Subsystem1/CopyRight2 ==

== system SF013A_PullCmpActv/PullCmpActv/PullCmpActvPer2/PullCmpActvPer2/LongTermErrIntgtr /If Action Subsystem1/If Action Subsystem/CopyRight2 ==

== system SF013A_PullCmpActv/PullCmpActv/PullCmpActvPer2/PullCmpActvPer2/LongTermErrIntgtr /If Action Subsystem1/If Action Subsystem1/CopyRight2 ==

== system SF013A_PullCmpActv/PullCmpActv/PullCmpActvPer1/PullCmpActvPer1/ActvCmpEna/ElapsedTime/If true and last step is true calculate elapsed time /GetTiSpan100MicroSec32bit/CopyRight2 ==
